simulink model "Thesis"  (R2021b)
settings: Solver=ode1  StartTime=0.0  StopTime=75  FixedStep=0.01  RelTol=1e-3
values from neighbouring files (symbols this model uses):
  hf_kJ_kg_ = [0.9007 9.2488 17.5909 25.9279 34.2606 42.5897 50.916 59.2401 67.5625 75.8837 84.2043 92.5247 ... (71 elements, 71x1)]    [thesis_workspace.mat]
  hfg_kJ_kg_ = [2499.12 2495.15 2491.01 2486.72 2482.31 2477.83 2473.27 2468.66 2464.02 2459.34 2454.65 2449.94 ... (71 elements, 71x1)]    [thesis_workspace.mat]
  hfg_kJ_kg_flip = [2144.27 2150.26 2156.21 2162.11 2167.98 2173.8 2179.58 2185.33 2191.04 2196.71 2202.35 2207.95 ... (71 elements, 71x1)]    [thesis_workspace.mat]
  hg_kJ_kg_ = [2500.02 2504.4 2508.6 2512.64 2516.58 2520.42 2524.19 2527.9 2531.58 2535.23 2538.85 2542.46 ... (71 elements, 71x1)]    [thesis_workspace.mat]
  Psat_kPa_ = [0.6119 0.7066 0.814 0.9357 1.0732 1.2282 1.4026 1.5985 1.818 2.0635 2.3376 2.6431 ... (71 elements, 71x1)]    [thesis_workspace.mat]
  Psat_kPa_flip = [361.402 341.408 322.317 304.097 286.72 270.156 254.377 239.354 225.062 211.472 198.559 186.297 ... (71 elements, 71x1)]    [thesis_workspace.mat]
  sf_kJ_kg_ = [-0.0013 0.0297 0.0604 0.0908 0.1209 0.1508 0.1804 0.2098 0.2389 0.2678 0.2964 0.3249 ... (71 elements, 71x1)]    [thesis_workspace.mat]
  sfg_kJ_kg_ = [9.1595 9.0755 8.9928 8.9113 8.8309 8.7518 8.6738 8.5969 8.5211 8.4463 8.3725 8.2998 ... (71 elements, 71x1)]    [thesis_workspace.mat]
  sg_kJ_kg_ = [9.1582 9.1052 9.0531 9.002 8.9519 8.9026 8.8542 8.8066 8.7599 8.7141 8.669 8.6247 ... (71 elements, 71x1)]    [thesis_workspace.mat]
  T_C_ = [0 2 4 6 8 10 12 14 16 18 20 22 ... (71 elements, 71x1)]    [thesis_workspace.mat]
  uf_kJ_kg_ = [0.9001 9.2481 17.5901 25.9269 34.2595 42.5885 50.9146 59.2385 67.5607 75.8817 84.202 92.522 ... (71 elements, 71x1)]    [thesis_workspace.mat]
  ufg_kJ_kg_ = [2373.12 2368.24 2363.17 2357.97 2352.66 2347.25 2341.79 2336.27 2330.71 2325.13 2319.53 2313.91 ... (71 elements, 71x1)]    [thesis_workspace.mat]
  ug_kJ_kg_ = [2374.02 2377.48 2380.76 2383.9 2386.91 2389.84 2392.7 2395.51 2398.27 2401.01 2403.73 2406.43 ... (71 elements, 71x1)]    [thesis_workspace.mat]
  vf_m3_kg_ = [0.000995 0.000995 0.000996 0.000996 0.000997 0.000997 0.000998 0.000999 0.000999 0.001 0.001 0.001001 ... (71 elements, 71x1)]    [thesis_workspace.mat]
  vfg_m3_kg_ = [205.93 179.63 157.04 137.59 120.82 106.31 93.74 82.83 73.33 65.04 57.8 51.46 ... (71 elements, 71x1)]    [thesis_workspace.mat]
  vg_m3_kg_ = [205.94 179.63 157.04 137.59 120.82 106.31 93.74 82.83 73.33 65.04 57.8 51.47 ... (71 elements, 71x1)]    [thesis_workspace.mat]
libraries: simulink x3, slpidlib x2
settings Model: Creator=mluser  LastModifiedBy=mluser

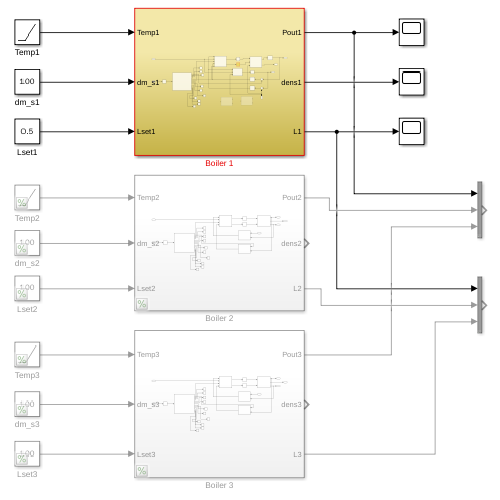
[thumbnail: Simulink's stored preview of the top-level diagram]
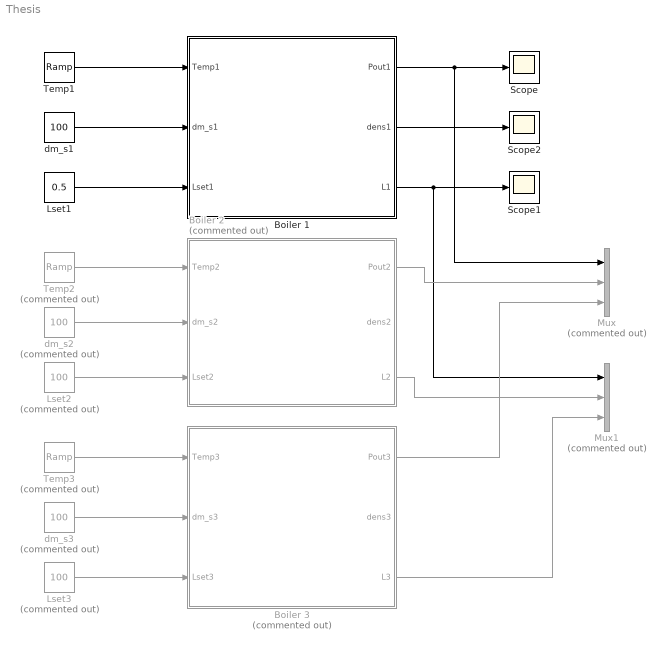
== system Thesis ==
  Boiler 1 : Subsystem
  Boiler 2 : Subsystem  Commented=on
  Boiler 3 : Subsystem  Commented=on
  Lset1 : Constant  Value=0.5
  Lset2 : Constant  Commented=on  Value=100
  Lset3 : Constant  Commented=on  Value=100
  Mux : Mux  Commented=on  Inputs=3
  Mux1 : Mux  Commented=on  Inputs=3
  Scope : Scope
  Scope1 : Scope
  Scope2 : Scope
  Temp1 : simulink/Sources/Ramp  slope=2  start=1  InitialOutput=1
  Temp2 : simulink/Sources/Ramp  Commented=on  slope=2  start=0  InitialOutput=0
  Temp3 : simulink/Sources/Ramp  Commented=on  slope=2  start=0  InitialOutput=0
  dm_s1 : Constant  Value=100
  dm_s2 : Constant  Commented=on  Value=100
  dm_s3 : Constant  Commented=on  Value=100
  wires:
  Temp1/1 -> Boiler 1/1(Temp1)
  dm_s1/1 -> Boiler 1/2(dm_s1)
  Temp2/1 -> Boiler 2/1(Temp2)
  dm_s2/1 -> Boiler 2/2(dm_s2)
  Temp3/1 -> Boiler 3/1(Temp3)
  dm_s3/1 -> Boiler 3/2(dm_s3)
  Lset1/1 -> Boiler 1/3(Lset1)
  Lset2/1 -> Boiler 2/3(Lset2)
  Lset3/1 -> Boiler 3/3(Lset3)
  Boiler 1/1(Pout1) -> Mux/1, Scope/1
  Boiler 1/3(L1) -> Mux1/1, Scope1/1
  Boiler 1/2(dens1) -> Scope2/1
  Boiler 2/1(Pout2) -> Mux/2
  Boiler 3/1(Pout3) -> Mux/3
  Boiler 2/3(L2) -> Mux1/2
  Boiler 3/3(L3) -> Mux1/3

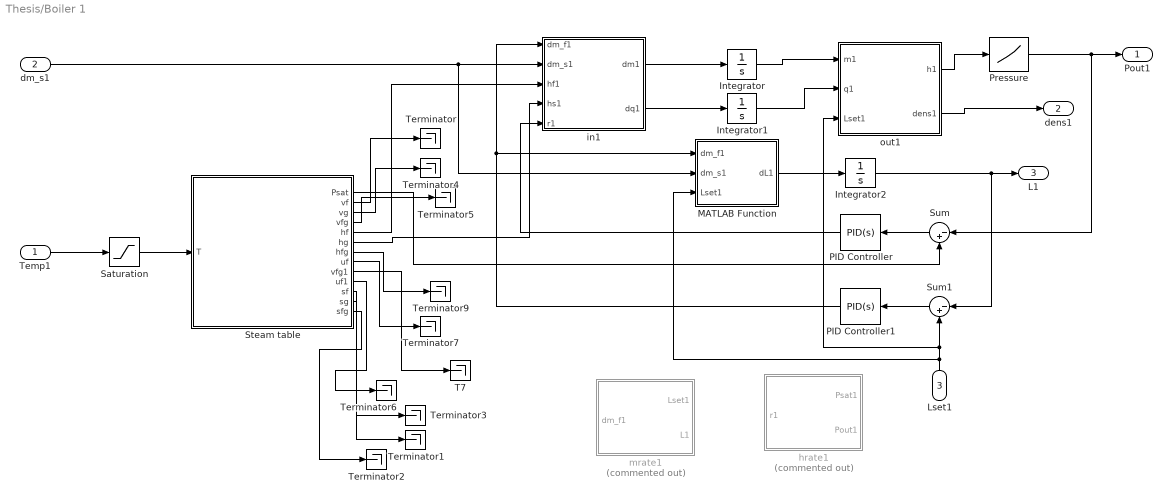
== system Thesis/Boiler 1 ==
  Temp1 : Inport
  dm_s1 : Inport  Port=2
  Lset1 : Inport  Port=3
  Integrator : Integrator
  Integrator1 : Integrator  InitialCondition=1
  Integrator2 : Integrator
  MATLAB Function : MATLAB Function  TreatAsAtomicUnit=on
  PID Controller : slpidlib/PID Controller  Controller=PID  Form=Parallel  TimeDomain=Continuous-time  UseExternalTs=off  SampleTime=-1  IntegratorMethod=Forward Euler  FilterMethod=Forward Euler  ControllerParametersSource=internal  P=25  I=0  D=0  UseFilter=on  N=100  TunerSelectOption=Transfer Function Based (PID Tuner App)  InitialConditionSource=internal  InitialConditionForIntegrator=0  InitialConditionForFilter=0  DifferentiatorICPrevScaledInput=0  ExternalReset=none  TrackingMode=off  Kt=1  LimitOutput=off  SatLimitsSource=internal  UpperSaturationLimit=inf  LowerSaturationLimit=-inf  LinearizeAsGain=on  AntiWindupMode=none  Kb=1  POutMin=[]  POutMax=[]  IOutMin=[]  IOutMax=[]  DOutMin=[]  DOutMax=[]  NOutMin=[]  NOutMax=[]  SumOutMin=[]  SumOutMax=[]  SaturationOutMin=[]  SaturationOutMax=[]  PParamMin=[]  PParamMax=[]  IParamMin=[]  IParamMax=[]  DParamMin=[]  DParamMax=[]  NParamMin=[]  NParamMax=[]  KbParamMin=[]  KbParamMax=[]  KtParamMin=[]  KtParamMax=[]  KbOutMin=[]  KbOutMax=[]  KtOutMin=[]  KtOutMax=[]  IntegratorOutMin=[]  IntegratorOutMax=[]  FilterOutMin=[]  FilterOutMax=[]  SumI1OutMin=[]  SumI1OutMax=[]  SumI2OutMin=[]  SumI2OutMax=[]  SumI3OutMin=[]  SumI3OutMax=[]  SumI4OutMin=[]  SumI4OutMax=[]  SumDOutMin=[]  SumDOutMax=[]  DifferentiatorOutMin=[]  DifferentiatorOutMax=[]  FilterDiffOutCoefMin=[]  FilterDiffOutCoefMax=[]  ReciprocalOutMin=[]  ReciprocalOutMax=[]  SumDenOutMin=[]  SumDenOutMax=[]  SumNumOutMin=[]  SumNumOutMax=[]  DivideOutMin=[]  DivideOutMax=[]  UdiffTsProdOutMin=[]  UdiffTsProdOutMax=[]  NTsProdOutMin=[]  NTsProdOutMax=[]  UintegralTsProdOutMin=[]  UintegralTsProdOutMax=[]  UngainTsProdOutMin=[]  UngainTsProdOutMax=[]  IntegratorContinuousStateAttributes=''  IntegratorStateMustResolveToSignalObject=off  IntegratorRTWStateStorageClass=Auto  FilterContinuousStateAttributes=''  FilterStateMustResolveToSignalObject=off  FilterRTWStateStorageClass=Auto  ParallelPVariant=InternalParameters  IdealPVariant=Disabled  IVariant=InternalParameters  DVariant=InternalParameters  IntegratorVariant=Continuous  SatVariant=Disabled  AWVariant=Passthrough  PCopyVariant=Disabled  TRVariant=Disabled  FdbkBlocksVariant=Forward  IdealPFdbkVariant=Disabled  SatFdbkVariant=Disabled  DerivativeFilterVariant=ContFilter  NVariant=InternalParameters  NCopyVariant=Disabled  FilterICVariant=InternalICsFilter  IntegratorICVariant=InternalICs  ExternalResetVariant=Disabled  TRSumVariant=Passthrough  SumFdbkVariant=Disabled  SumVariant=Sum_PID  TsampFilterVariant=InternalTs  TsampNgainVariant=Passthrough  TsampIntegralVariant=Passthrough  ExternalSaturationOutDataTypeStr=Inherit: Same as second input
  PID Controller1 : slpidlib/PID Controller  Controller=PID  Form=Parallel  TimeDomain=Continuous-time  UseExternalTs=off  SampleTime=-1  IntegratorMethod=Forward Euler  FilterMethod=Forward Euler  ControllerParametersSource=internal  P=25  I=0  D=0  UseFilter=on  N=100  TunerSelectOption=Transfer Function Based (PID Tuner App)  InitialConditionSource=internal  InitialConditionForIntegrator=0  InitialConditionForFilter=0  DifferentiatorICPrevScaledInput=0  ExternalReset=none  TrackingMode=off  Kt=1  LimitOutput=off  SatLimitsSource=internal  UpperSaturationLimit=inf  LowerSaturationLimit=-inf  LinearizeAsGain=on  AntiWindupMode=none  Kb=1  POutMin=[]  POutMax=[]  IOutMin=[]  IOutMax=[]  DOutMin=[]  DOutMax=[]  NOutMin=[]  NOutMax=[]  SumOutMin=[]  SumOutMax=[]  SaturationOutMin=[]  SaturationOutMax=[]  PParamMin=[]  PParamMax=[]  IParamMin=[]  IParamMax=[]  DParamMin=[]  DParamMax=[]  NParamMin=[]  NParamMax=[]  KbParamMin=[]  KbParamMax=[]  KtParamMin=[]  KtParamMax=[]  KbOutMin=[]  KbOutMax=[]  KtOutMin=[]  KtOutMax=[]  IntegratorOutMin=[]  IntegratorOutMax=[]  FilterOutMin=[]  FilterOutMax=[]  SumI1OutMin=[]  SumI1OutMax=[]  SumI2OutMin=[]  SumI2OutMax=[]  SumI3OutMin=[]  SumI3OutMax=[]  SumI4OutMin=[]  SumI4OutMax=[]  SumDOutMin=[]  SumDOutMax=[]  DifferentiatorOutMin=[]  DifferentiatorOutMax=[]  FilterDiffOutCoefMin=[]  FilterDiffOutCoefMax=[]  ReciprocalOutMin=[]  ReciprocalOutMax=[]  SumDenOutMin=[]  SumDenOutMax=[]  SumNumOutMin=[]  SumNumOutMax=[]  DivideOutMin=[]  DivideOutMax=[]  UdiffTsProdOutMin=[]  UdiffTsProdOutMax=[]  NTsProdOutMin=[]  NTsProdOutMax=[]  UintegralTsProdOutMin=[]  UintegralTsProdOutMax=[]  UngainTsProdOutMin=[]  UngainTsProdOutMax=[]  IntegratorContinuousStateAttributes=''  IntegratorStateMustResolveToSignalObject=off  IntegratorRTWStateStorageClass=Auto  FilterContinuousStateAttributes=''  FilterStateMustResolveToSignalObject=off  FilterRTWStateStorageClass=Auto  ParallelPVariant=InternalParameters  IdealPVariant=Disabled  IVariant=InternalParameters  DVariant=InternalParameters  IntegratorVariant=Continuous  SatVariant=Disabled  AWVariant=Passthrough  PCopyVariant=Disabled  TRVariant=Disabled  FdbkBlocksVariant=Forward  IdealPFdbkVariant=Disabled  SatFdbkVariant=Disabled  DerivativeFilterVariant=ContFilter  NVariant=InternalParameters  NCopyVariant=Disabled  FilterICVariant=InternalICsFilter  IntegratorICVariant=InternalICs  ExternalResetVariant=Disabled  TRSumVariant=Passthrough  SumFdbkVariant=Disabled  SumVariant=Sum_PID  TsampFilterVariant=InternalTs  TsampNgainVariant=Passthrough  TsampIntegralVariant=Passthrough  ExternalSaturationOutDataTypeStr=Inherit: Same as second input
  Pressure : Lookup_n-D  NumberOfTableDimensions=1  BreakpointsForDimension1=hfg_kJ_kg_flip  Table=Psat_kPa_flip  InternalRulePriority=Speed  RndMeth=Simplest  InputSameDT=on
  Saturation : Saturate  UpperLimit=50  LowerLimit=0
  "Steam table " : Subsystem
  Sum : Sum  Inputs=|-+
  Sum1 : Sum  Inputs=|-+
  T7 : Terminator
  Terminator{,1..7,9} (9 alike) : Terminator
  hrate1 : MATLAB Function  Commented=on  TreatAsAtomicUnit=on
  in1 : MATLAB Function  TreatAsAtomicUnit=on
  mrate1 : MATLAB Function  Commented=on  TreatAsAtomicUnit=on
  out1 : MATLAB Function  TreatAsAtomicUnit=on
  Pout1 : Outport
  dens1 : Outport  Port=2
  L1 : Outport  Port=3
  wires:
  "Steam table "/12(sg) -> Terminator1/1
  "Steam table "/13(sfg) -> Terminator2/1
  "Steam table "/3(vg) -> Terminator4/1
  "Steam table "/6(hg) -> in1/4(hs1)
  "Steam table "/7(hfg) -> Terminator9/1
  in1/1(dm1) -> Integrator/1
  Temp1/1 -> Saturation/1
  "Steam table "/2(vf) -> Terminator/1
  dm_s1/1 -> MATLAB Function/2(dm_s1), in1/2(dm_s1)
  "Steam table "/10(uf1) -> Terminator6/1
  "Steam table "/8(uf) -> Terminator7/1
  Integrator/1 -> out1/1(m1)
  in1/2(dq1) -> Integrator1/1
  "Steam table "/9(vfg1) -> T7/1
  Integrator1/1 -> out1/2(q1)
  "Steam table "/11(sf) -> Terminator3/1
  out1/2(dens1) -> dens1/1
  out1/1(h1) -> Pressure/1
  Pressure/1 -> Sum/1, Pout1/1
  Sum/1 -> PID Controller/1
  PID Controller/1 -> in1/5(r1)
  "Steam table "/1(Psat) -> Sum/2
  Sum1/1 -> PID Controller1/1
  PID Controller1/1 -> MATLAB Function/1(dm_f1), in1/1(dm_f1)
  Lset1/1 -> Sum1/2, out1/3(Lset1), MATLAB Function/3(Lset1)
  "Steam table "/4(vfg) -> Terminator5/1
  "Steam table "/5(hf) -> in1/3(hf1)
  Integrator2/1 -> Sum1/1, L1/1
  MATLAB Function/1(dL1) -> Integrator2/1
  Saturation/1 -> "Steam table "/1(T)

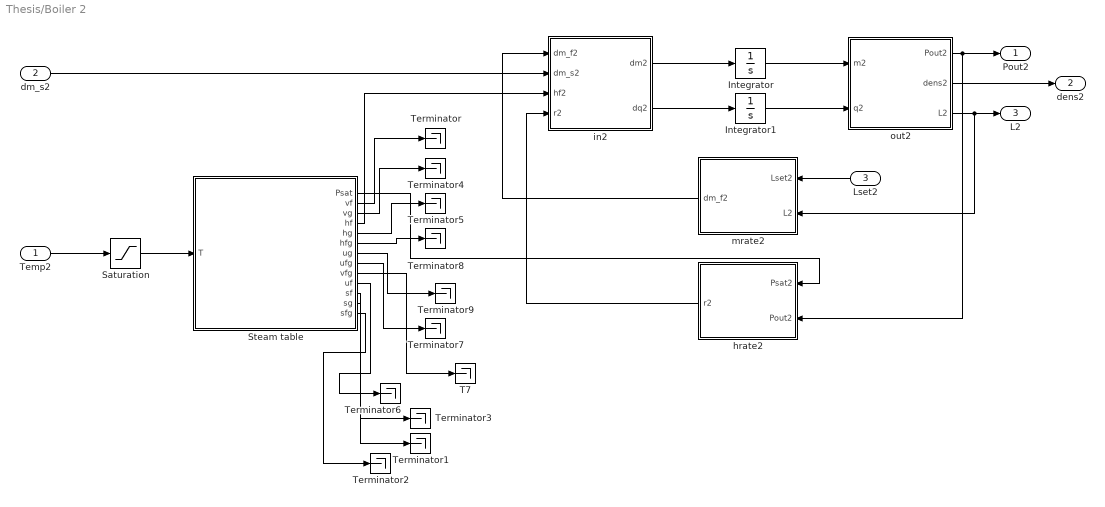
== system Thesis/Boiler 2 ==
  Temp2 : Inport
  dm_s2 : Inport  Port=2
  Lset2 : Inport  Port=3
  Integrator : Integrator
  Integrator1 : Integrator
  Saturation : Saturate  UpperLimit=50  LowerLimit=0
  "Steam table " : Subsystem
  T7 : Terminator
  Terminator{,1..9} (10 alike) : Terminator
  hrate2 : MATLAB Function  TreatAsAtomicUnit=on
  in2 : MATLAB Function  TreatAsAtomicUnit=on
  mrate2 : MATLAB Function  TreatAsAtomicUnit=on
  out2 : MATLAB Function  TreatAsAtomicUnit=on
  Pout2 : Outport
  dens2 : Outport  Port=2
  L2 : Outport  Port=3
  wires:
  "Steam table "/12(sg) -> Terminator1/1
  "Steam table "/13(sfg) -> Terminator2/1
  out2/1(Pout2) -> Pout2/1, hrate2/2(Pout2)
  out2/3(L2) -> L2/1, mrate2/2(L2)
  "Steam table "/3(vg) -> Terminator4/1
  "Steam table "/4(hf) -> in2/3(hf2)
  "Steam table "/6(hfg) -> Terminator8/1
  "Steam table "/7(ug) -> Terminator9/1
  in2/1(dm2) -> Integrator/1
  Temp2/1 -> Saturation/1
  hrate2/1(r2) -> in2/4(r2)
  "Steam table "/2(vf) -> Terminator/1
  "Steam table "/1(Psat) -> hrate2/1(Psat2)
  dm_s2/1 -> in2/2(dm_s2)
  "Steam table "/5(hg) -> Terminator5/1
  "Steam table "/10(uf) -> Terminator6/1
  "Steam table "/8(ufg) -> Terminator7/1
  mrate2/1(dm_f2) -> in2/1(dm_f2)
  Integrator/1 -> out2/1(m2)
  in2/2(dq2) -> Integrator1/1
  "Steam table "/9(vfg) -> T7/1
  Integrator1/1 -> out2/2(q2)
  Saturation/1 -> "Steam table "/1(T)
  "Steam table "/11(sf) -> Terminator3/1
  Lset2/1 -> mrate2/1(Lset2)
  out2/2(dens2) -> dens2/1

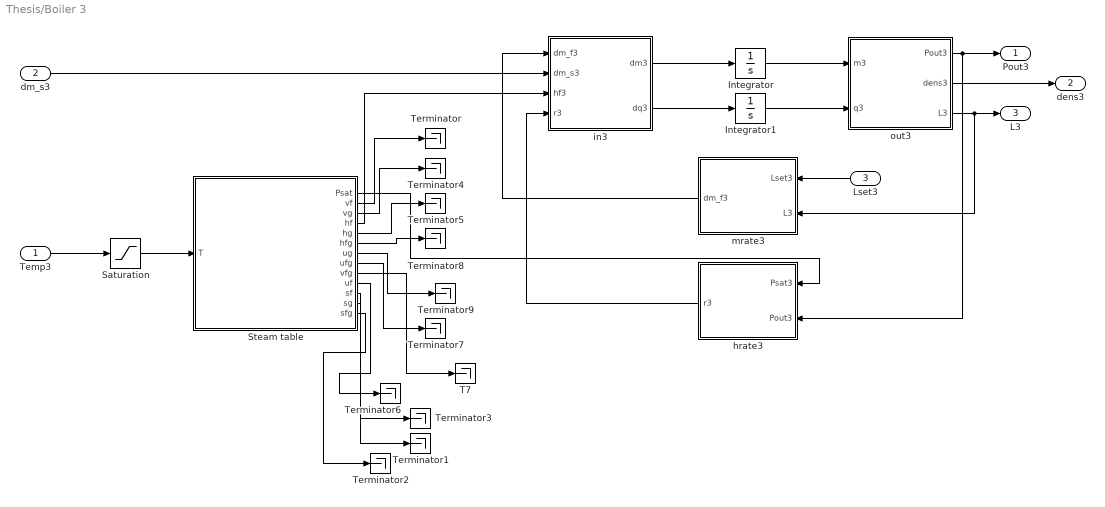
== system Thesis/Boiler 3 ==
  Temp3 : Inport
  dm_s3 : Inport  Port=2
  Lset3 : Inport  Port=3
  Integrator : Integrator
  Integrator1 : Integrator
  Saturation : Saturate  UpperLimit=50  LowerLimit=0
  "Steam table " : Subsystem
  T7 : Terminator
  Terminator{,1..9} (10 alike) : Terminator
  hrate3 : MATLAB Function  TreatAsAtomicUnit=on
  in3 : MATLAB Function  TreatAsAtomicUnit=on
  mrate3 : MATLAB Function  TreatAsAtomicUnit=on
  out3 : MATLAB Function  TreatAsAtomicUnit=on
  Pout3 : Outport
  dens3 : Outport  Port=2
  L3 : Outport  Port=3
  wires:
  "Steam table "/12(sg) -> Terminator1/1
  "Steam table "/13(sfg) -> Terminator2/1
  out3/1(Pout3) -> Pout3/1, hrate3/2(Pout3)
  out3/3(L3) -> L3/1, mrate3/2(L3)
  "Steam table "/3(vg) -> Terminator4/1
  "Steam table "/4(hf) -> in3/3(hf3)
  "Steam table "/6(hfg) -> Terminator8/1
  "Steam table "/7(ug) -> Terminator9/1
  in3/1(dm3) -> Integrator/1
  Temp3/1 -> Saturation/1
  hrate3/1(r3) -> in3/4(r3)
  "Steam table "/2(vf) -> Terminator/1
  "Steam table "/1(Psat) -> hrate3/1(Psat3)
  dm_s3/1 -> in3/2(dm_s3)
  "Steam table "/5(hg) -> Terminator5/1
  "Steam table "/10(uf) -> Terminator6/1
  "Steam table "/8(ufg) -> Terminator7/1
  mrate3/1(dm_f3) -> in3/1(dm_f3)
  Integrator/1 -> out3/1(m3)
  in3/2(dq3) -> Integrator1/1
  "Steam table "/9(vfg) -> T7/1
  Integrator1/1 -> out3/2(q3)
  Saturation/1 -> "Steam table "/1(T)
  "Steam table "/11(sf) -> Terminator3/1
  Lset3/1 -> mrate3/1(Lset3)
  out3/2(dens3) -> dens3/1

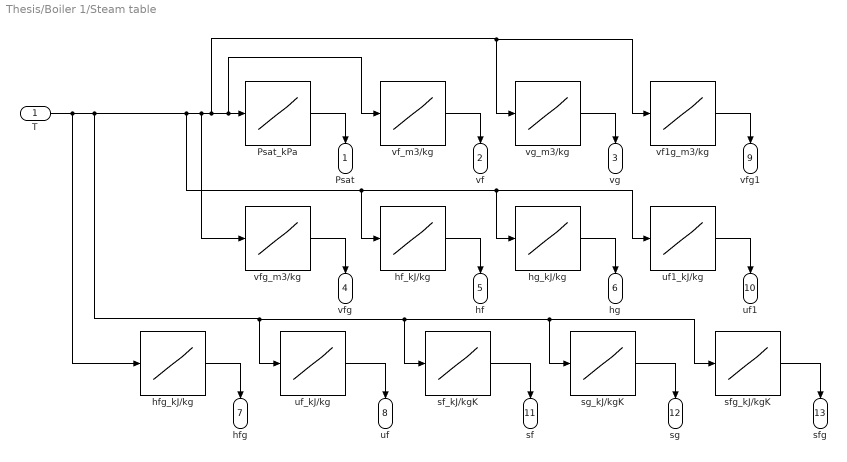
== system Thesis/Boiler 1/Steam table  ==
  T : Inport
  Psat_kPa : Lookup_n-D  NumberOfTableDimensions=1  BreakpointsForDimension1=T_C_  Table=Psat_kPa_  InternalRulePriority=Speed  RndMeth=Simplest  InputSameDT=on
  hf_kJ/kg : Lookup_n-D  NumberOfTableDimensions=1  BreakpointsForDimension1=T_C_  Table=hg_kJ_kg_  InternalRulePriority=Speed  RndMeth=Simplest  InputSameDT=on
  hfg_kJ/kg : Lookup_n-D  NumberOfTableDimensions=1  BreakpointsForDimension1=T_C_  Table=hfg_kJ_kg_  InternalRulePriority=Speed  RndMeth=Simplest  InputSameDT=on
  hg_kJ/kg : Lookup_n-D  NumberOfTableDimensions=1  BreakpointsForDimension1=T_C_  Table=hfg_kJ_kg_  InternalRulePriority=Speed  RndMeth=Simplest  InputSameDT=on
  sf_kJ/kgK : Lookup_n-D  NumberOfTableDimensions=1  BreakpointsForDimension1=T_C_  Table=sf_kJ_kg_  InternalRulePriority=Speed  RndMeth=Simplest  InputSameDT=on
  sfg_kJ/kgK : Lookup_n-D  NumberOfTableDimensions=1  BreakpointsForDimension1=T_C_  Table=sfg_kJ_kg_  InternalRulePriority=Speed  RndMeth=Simplest  InputSameDT=on
  sg_kJ/kgK : Lookup_n-D  NumberOfTableDimensions=1  BreakpointsForDimension1=T_C_  Table=sg_kJ_kg_  InternalRulePriority=Speed  RndMeth=Simplest  InputSameDT=on
  uf1_kJ/kg : Lookup_n-D  NumberOfTableDimensions=1  BreakpointsForDimension1=T_C_  Table=ufg_kJ_kg_  InternalRulePriority=Speed  RndMeth=Simplest  InputSameDT=on
  uf_kJ/kg : Lookup_n-D  NumberOfTableDimensions=1  BreakpointsForDimension1=T_C_  Table=uf_kJ_kg_  InternalRulePriority=Speed  RndMeth=Simplest  InputSameDT=on
  vf1g_m3/kg : Lookup_n-D  NumberOfTableDimensions=1  BreakpointsForDimension1=T_C_  Table=ug_kJ_kg_  InternalRulePriority=Speed  RndMeth=Simplest  InputSameDT=on
  vf_m3/kg : Lookup_n-D  NumberOfTableDimensions=1  BreakpointsForDimension1=T_C_  Table=vf_m3_kg_  InternalRulePriority=Speed  RndMeth=Simplest  InputSameDT=on
  vfg_m3/kg : Lookup_n-D  NumberOfTableDimensions=1  BreakpointsForDimension1=T_C_  Table=vfg_m3_kg_  InternalRulePriority=Speed  RndMeth=Simplest  InputSameDT=on
  vg_m3/kg : Lookup_n-D  NumberOfTableDimensions=1  BreakpointsForDimension1=T_C_  Table=vg_m3_kg_  InternalRulePriority=Speed  RndMeth=Simplest  InputSameDT=on
  Psat : Outport
  vf : Outport  Port=2
  vg : Outport  Port=3
  vfg : Outport  Port=4
  hf : Outport  Port=5
  hg : Outport  Port=6
  hfg : Outport  Port=7
  uf : Outport  Port=8
  vfg1 : Outport  Port=9
  uf1 : Outport  Port=10
  sf : Outport  Port=11
  sg : Outport  Port=12
  sfg : Outport  Port=13
  wires:
  uf_kJ/kg/1 -> uf/1
  hg_kJ/kg/1 -> hg/1
  uf1_kJ/kg/1 -> uf1/1
  vfg_m3/kg/1 -> vfg/1
  sg_kJ/kgK/1 -> sg/1
  vg_m3/kg/1 -> vg/1
  hfg_kJ/kg/1 -> hfg/1
  T/1 -> sfg_kJ/kgK/1, sg_kJ/kgK/1, sf_kJ/kgK/1, uf_kJ/kg/1, uf1_kJ/kg/1, hg_kJ/kg/1, hf_kJ/kg/1, vfg_m3/kg/1, vf1g_m3/kg/1, vg_m3/kg/1, vf_m3/kg/1, Psat_kPa/1, hfg_kJ/kg/1
  sfg_kJ/kgK/1 -> sfg/1
  hf_kJ/kg/1 -> hf/1
  vf1g_m3/kg/1 -> vfg1/1
  sf_kJ/kgK/1 -> sf/1
  Psat_kPa/1 -> Psat/1
  vf_m3/kg/1 -> vf/1

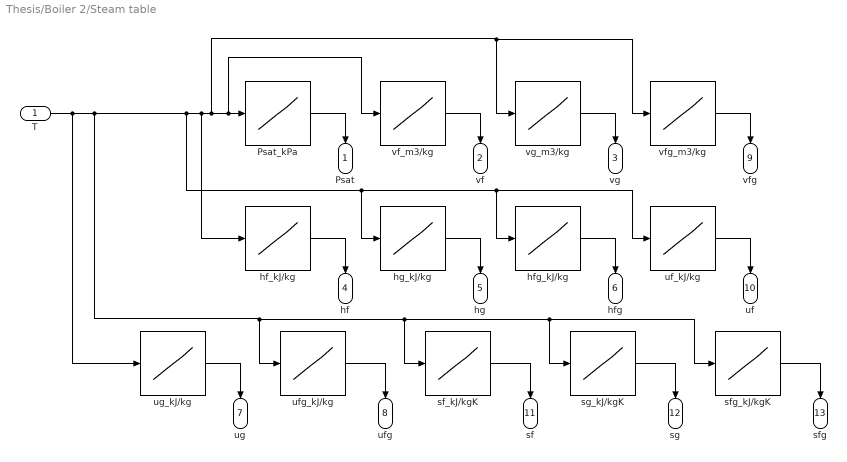
== system Thesis/Boiler 2/Steam table  ==
  T : Inport
  Psat_kPa : Lookup_n-D  NumberOfTableDimensions=1  BreakpointsForDimension1=T_C_  Table=Psat_kPa_  InternalRulePriority=Speed  RndMeth=Simplest  InputSameDT=on
  hf_kJ/kg : Lookup_n-D  NumberOfTableDimensions=1  BreakpointsForDimension1=T_C_  Table=vfg_m3_kg_  InternalRulePriority=Speed  RndMeth=Simplest  InputSameDT=on
  hfg_kJ/kg : Lookup_n-D  NumberOfTableDimensions=1  BreakpointsForDimension1=T_C_  Table=hg_kJ_kg_  InternalRulePriority=Speed  RndMeth=Simplest  InputSameDT=on
  hg_kJ/kg : Lookup_n-D  NumberOfTableDimensions=1  BreakpointsForDimension1=T_C_  Table=hf_kJ_kg_  InternalRulePriority=Speed  RndMeth=Simplest  InputSameDT=on
  sf_kJ/kgK : Lookup_n-D  NumberOfTableDimensions=1  BreakpointsForDimension1=T_C_  Table=sf_kJ_kg_  InternalRulePriority=Speed  RndMeth=Simplest  InputSameDT=on
  sfg_kJ/kgK : Lookup_n-D  NumberOfTableDimensions=1  BreakpointsForDimension1=T_C_  Table=sfg_kJ_kg_  InternalRulePriority=Speed  RndMeth=Simplest  InputSameDT=on
  sg_kJ/kgK : Lookup_n-D  NumberOfTableDimensions=1  BreakpointsForDimension1=T_C_  Table=sg_kJ_kg_  InternalRulePriority=Speed  RndMeth=Simplest  InputSameDT=on
  uf_kJ/kg : Lookup_n-D  NumberOfTableDimensions=1  BreakpointsForDimension1=T_C_  Table=ufg_kJ_kg_  InternalRulePriority=Speed  RndMeth=Simplest  InputSameDT=on
  ufg_kJ/kg : Lookup_n-D  NumberOfTableDimensions=1  BreakpointsForDimension1=T_C_  Table=uf_kJ_kg_  InternalRulePriority=Speed  RndMeth=Simplest  InputSameDT=on
  ug_kJ/kg : Lookup_n-D  NumberOfTableDimensions=1  BreakpointsForDimension1=T_C_  Table=hfg_kJ_kg_  InternalRulePriority=Speed  RndMeth=Simplest  InputSameDT=on
  vf_m3/kg : Lookup_n-D  NumberOfTableDimensions=1  BreakpointsForDimension1=T_C_  Table=vf_m3_kg_  InternalRulePriority=Speed  RndMeth=Simplest  InputSameDT=on
  vfg_m3/kg : Lookup_n-D  NumberOfTableDimensions=1  BreakpointsForDimension1=T_C_  Table=ug_kJ_kg_  InternalRulePriority=Speed  RndMeth=Simplest  InputSameDT=on
  vg_m3/kg : Lookup_n-D  NumberOfTableDimensions=1  BreakpointsForDimension1=T_C_  Table=vg_m3_kg_  InternalRulePriority=Speed  RndMeth=Simplest  InputSameDT=on
  Psat : Outport
  vf : Outport  Port=2
  vg : Outport  Port=3
  hf : Outport  Port=4
  hg : Outport  Port=5
  hfg : Outport  Port=6
  ug : Outport  Port=7
  ufg : Outport  Port=8
  vfg : Outport  Port=9
  uf : Outport  Port=10
  sf : Outport  Port=11
  sg : Outport  Port=12
  sfg : Outport  Port=13
  wires:
  ufg_kJ/kg/1 -> ufg/1
  hfg_kJ/kg/1 -> hfg/1
  uf_kJ/kg/1 -> uf/1
  hf_kJ/kg/1 -> hf/1
  sg_kJ/kgK/1 -> sg/1
  vg_m3/kg/1 -> vg/1
  ug_kJ/kg/1 -> ug/1
  T/1 -> sfg_kJ/kgK/1, sg_kJ/kgK/1, sf_kJ/kgK/1, ufg_kJ/kg/1, uf_kJ/kg/1, hfg_kJ/kg/1, hg_kJ/kg/1, hf_kJ/kg/1, vfg_m3/kg/1, vg_m3/kg/1, vf_m3/kg/1, Psat_kPa/1, ug_kJ/kg/1
  sfg_kJ/kgK/1 -> sfg/1
  hg_kJ/kg/1 -> hg/1
  vfg_m3/kg/1 -> vfg/1
  sf_kJ/kgK/1 -> sf/1
  Psat_kPa/1 -> Psat/1
  vf_m3/kg/1 -> vf/1

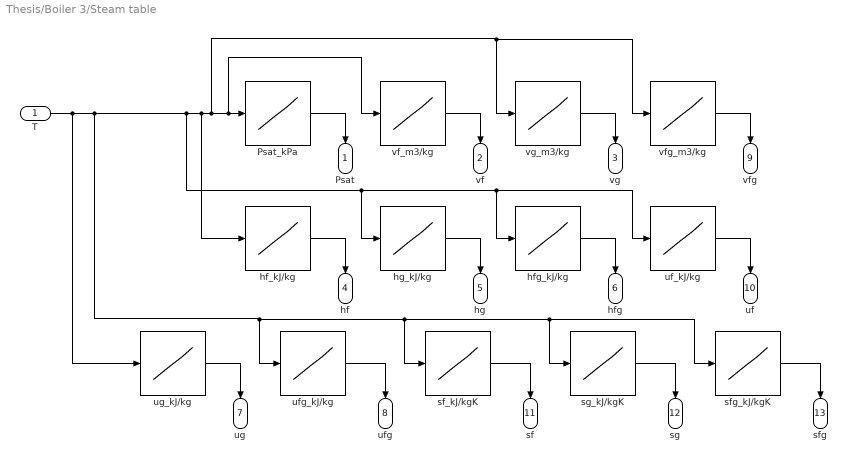
== system Thesis/Boiler 3/Steam table  ==
  T : Inport
  Psat_kPa : Lookup_n-D  NumberOfTableDimensions=1  BreakpointsForDimension1=T_C_  Table=Psat_kPa_  InternalRulePriority=Speed  RndMeth=Simplest  InputSameDT=on
  hf_kJ/kg : Lookup_n-D  NumberOfTableDimensions=1  BreakpointsForDimension1=T_C_  Table=vfg_m3_kg_  InternalRulePriority=Speed  RndMeth=Simplest  InputSameDT=on
  hfg_kJ/kg : Lookup_n-D  NumberOfTableDimensions=1  BreakpointsForDimension1=T_C_  Table=hg_kJ_kg_  InternalRulePriority=Speed  RndMeth=Simplest  InputSameDT=on
  hg_kJ/kg : Lookup_n-D  NumberOfTableDimensions=1  BreakpointsForDimension1=T_C_  Table=hf_kJ_kg_  InternalRulePriority=Speed  RndMeth=Simplest  InputSameDT=on
  sf_kJ/kgK : Lookup_n-D  NumberOfTableDimensions=1  BreakpointsForDimension1=T_C_  Table=sf_kJ_kg_  InternalRulePriority=Speed  RndMeth=Simplest  InputSameDT=on
  sfg_kJ/kgK : Lookup_n-D  NumberOfTableDimensions=1  BreakpointsForDimension1=T_C_  Table=sfg_kJ_kg_  InternalRulePriority=Speed  RndMeth=Simplest  InputSameDT=on
  sg_kJ/kgK : Lookup_n-D  NumberOfTableDimensions=1  BreakpointsForDimension1=T_C_  Table=sg_kJ_kg_  InternalRulePriority=Speed  RndMeth=Simplest  InputSameDT=on
  uf_kJ/kg : Lookup_n-D  NumberOfTableDimensions=1  BreakpointsForDimension1=T_C_  Table=ufg_kJ_kg_  InternalRulePriority=Speed  RndMeth=Simplest  InputSameDT=on
  ufg_kJ/kg : Lookup_n-D  NumberOfTableDimensions=1  BreakpointsForDimension1=T_C_  Table=uf_kJ_kg_  InternalRulePriority=Speed  RndMeth=Simplest  InputSameDT=on
  ug_kJ/kg : Lookup_n-D  NumberOfTableDimensions=1  BreakpointsForDimension1=T_C_  Table=hfg_kJ_kg_  InternalRulePriority=Speed  RndMeth=Simplest  InputSameDT=on
  vf_m3/kg : Lookup_n-D  NumberOfTableDimensions=1  BreakpointsForDimension1=T_C_  Table=vf_m3_kg_  InternalRulePriority=Speed  RndMeth=Simplest  InputSameDT=on
  vfg_m3/kg : Lookup_n-D  NumberOfTableDimensions=1  BreakpointsForDimension1=T_C_  Table=ug_kJ_kg_  InternalRulePriority=Speed  RndMeth=Simplest  InputSameDT=on
  vg_m3/kg : Lookup_n-D  NumberOfTableDimensions=1  BreakpointsForDimension1=T_C_  Table=vg_m3_kg_  InternalRulePriority=Speed  RndMeth=Simplest  InputSameDT=on
  Psat : Outport
  vf : Outport  Port=2
  vg : Outport  Port=3
  hf : Outport  Port=4
  hg : Outport  Port=5
  hfg : Outport  Port=6
  ug : Outport  Port=7
  ufg : Outport  Port=8
  vfg : Outport  Port=9
  uf : Outport  Port=10
  sf : Outport  Port=11
  sg : Outport  Port=12
  sfg : Outport  Port=13
  wires:
  ufg_kJ/kg/1 -> ufg/1
  hfg_kJ/kg/1 -> hfg/1
  uf_kJ/kg/1 -> uf/1
  hf_kJ/kg/1 -> hf/1
  sg_kJ/kgK/1 -> sg/1
  vg_m3/kg/1 -> vg/1
  ug_kJ/kg/1 -> ug/1
  T/1 -> sfg_kJ/kgK/1, sg_kJ/kgK/1, sf_kJ/kgK/1, ufg_kJ/kg/1, uf_kJ/kg/1, hfg_kJ/kg/1, hg_kJ/kg/1, hf_kJ/kg/1, vfg_m3/kg/1, vg_m3/kg/1, vf_m3/kg/1, Psat_kPa/1, ug_kJ/kg/1
  sfg_kJ/kgK/1 -> sfg/1
  hg_kJ/kg/1 -> hg/1
  vfg_m3/kg/1 -> vfg/1
  sf_kJ/kgK/1 -> sf/1
  Psat_kPa/1 -> Psat/1
  vf_m3/kg/1 -> vf/1

== matlab function Thesis/Boiler 3/mrate3 ==
  data: Lset3 input; dm_f3 output; L3 input
function dm_f3 = mrate3(Lset3,L3)

y = u;

== matlab function Thesis/Boiler 3/out3 ==
  data: m3 input; Pout3 output; q3 input; dens3 output; L3 output
function [Pout3,dens3,L3] = out3(m3,q3)

y = u;

== matlab function Thesis/Boiler 1/out1 ==
  data: m1 input; h1 output; q1 input; dens1 output; Lset1 input
function [h1,dens1] = out1(m1,q1,Lset1)

R = 1;
l = 3;
dif = 1-(Lset1/R);

Vt = l.*((R*R).*acos(dif)-(R-Lset1).*sqrt(2*R*Lset1-(Lset1*Lset1)));
V = uint16(Vt);
V1 = V/2;
h1 = q1/m1;
dens1 = m1/V1;

end

== matlab function Thesis/Boiler 1/MATLAB Function ==
  data: dm_f1 input; dL1 output; dm_s1 input; Lset1 input
function dL1 = dL1(dm_f1,dm_s1,Lset1)

R = 1;
l = 3;
dL1 = (dm_f1 - dm_s1)./(2*l.*sqrt(2*R*Lset1 - (Lset1*Lset1)));

end

== matlab function Thesis/Boiler 1/in1 ==
  data: dm_f1 input; dm1 output; dm_s1 input; hf1 input; hs1 input; r1 input; dq1 output
function [dm1,dq1] = in1(dm_f1,dm_s1,hf1,hs1,r1)

dm1 = dm_f1 - dm_s1;
dq1 = r1 + (dm_f1.*hf1) - (dm_s1.*hs1);

end

== matlab function Thesis/Boiler 1/hrate1 ==
  data: Psat1 input; r1 output; Pout1 input
function r1 = hrate1(Psat1,Pout1)

y = u;

== matlab function Thesis/Boiler 1/mrate1 ==
  data: Lset1 input; dm_f1 output; L1 input
function dm_f1 = mrate1(Lset1,L1)

y = u;

== matlab function Thesis/Boiler 2/hrate2 ==
  data: Psat2 input; r2 output; Pout2 input
function r2 = hrate2(Psat2,Pout2)

y = u;

== matlab function Thesis/Boiler 2/in2 ==
  data: dm_f2 input; dm2 output; dm_s2 input; hf2 input; r2 input; dq2 output
function [dm2,dq2] = in2(dm_f2,dm_s2,hf2,r2)

y = u;

== matlab function Thesis/Boiler 2/mrate2 ==
  data: Lset2 input; dm_f2 output; L2 input
function dm_f2 = mrate2(Lset2,L2)

y = u;

== matlab function Thesis/Boiler 2/out2 ==
  data: m2 input; Pout2 output; q2 input; dens2 output; L2 output
function [Pout2,dens2,L2] = out2(m2,q2)

y = u;

== matlab function Thesis/Boiler 3/hrate3 ==
  data: Psat3 input; r3 output; Pout3 input
function r3 = hrate3(Psat3,Pout3)

y = u;

== matlab function Thesis/Boiler 3/in3 ==
  data: dm_f3 input; dm3 output; dm_s3 input; hf3 input; r3 input; dq3 output
function [dm3,dq3] = in3(dm_f3,dm_s3,hf3,r3)

y = u;
